simulink model "ironCub"  (Simulink 8.6)
settings: Solver=FixedStepAuto  StartTime=0.0  StopTime=config.simulationTime  FixedStep=config.Ts  RelTol=1e-3
InitFcn:
  | cd(fileparts(which(bdroot)));
  | initIronCub;
StopFcn:
  | visualizer_demo(time.Data,state.Data,config,desired_x_dx_ddx_dddx_CoM,jetsIntensitiesByWeight);
values from neighbouring files (symbols this model uses):
  config = struct    [initIronCub.m]
  ROBOT_DOF = config.ndof    [initIronCub.m]
libraries: WBToolboxLibrary x99
(part 2 of 2)

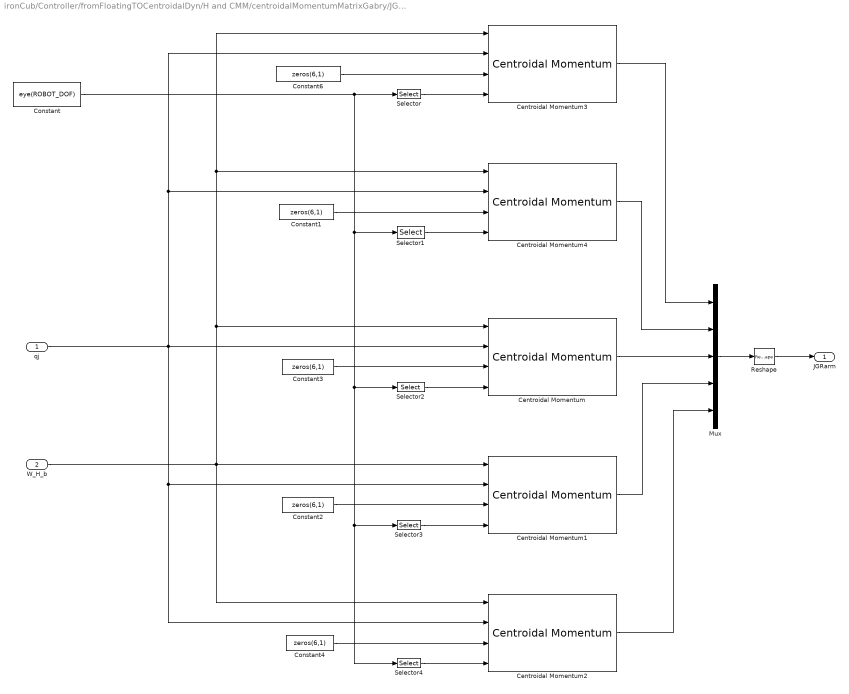
== system ironCub/Controller/fromFloatingTOCentroidalDyn/H and CMM/centroidalMomentumMatrixGabry/JGjoints/JGRarm ==
  qj : Inport
  W_H_b : Inport  Port=2
  Centroidal Momentum{,1..4} (5 alike) : WBToolboxLibrary/wholeBodyModel/Dynamics/Centroidal Momentum  robotName=WBT_robotName  localName=WBT_modelName  wbiFile=WBT_wbiFilename  wbiList=WBT_wbiList
  Constant : Constant  Value=eye(ROBOT_DOF)
  Constant{1..4,6} (5 alike) : Constant  Value=zeros(6,1)
  Mux : Mux  Inputs=5
  Reshape : Reshape  OutputDimensionality=Customize  OutputDimensions=[6,5]
  Selector : Selector  NumberOfDimensions=2  InputPortWidth=3  IndexOptions=Index vector (dialog),Select all  Indices=[9],1  OutputSizes=1,1
  Selector1 : Selector  NumberOfDimensions=2  InputPortWidth=3  IndexOptions=Index vector (dialog),Select all  Indices=[10],1  OutputSizes=1,1
  Selector2 : Selector  NumberOfDimensions=2  InputPortWidth=3  IndexOptions=Index vector (dialog),Select all  Indices=[11],1  OutputSizes=1,1
  Selector3 : Selector  NumberOfDimensions=2  InputPortWidth=3  IndexOptions=Index vector (dialog),Select all  Indices=[12],1  OutputSizes=1,1
  Selector4 : Selector  NumberOfDimensions=2  InputPortWidth=3  IndexOptions=Index vector (dialog),Select all  Indices=[13],1  OutputSizes=1,1
  JGRarm : Outport
  wires:
  Constant6/1 -> Centroidal Momentum3/3
  Constant1/1 -> Centroidal Momentum4/3
  Constant3/1 -> Centroidal Momentum/3
  Constant4/1 -> Centroidal Momentum2/3
  Constant2/1 -> Centroidal Momentum1/3
  qj/1 -> Centroidal Momentum4/2, Centroidal Momentum3/2, Centroidal Momentum2/2, Centroidal Momentum1/2, Centroidal Momentum/2
  W_H_b/1 -> Centroidal Momentum1/1, Centroidal Momentum2/1, Centroidal Momentum/1, Centroidal Momentum3/1, Centroidal Momentum4/1
  Constant/1 -> Selector4/1, Selector3/1, Selector2/1, Selector1/1, Selector/1
  Selector/1 -> Centroidal Momentum3/4
  Selector1/1 -> Centroidal Momentum4/4
  Selector2/1 -> Centroidal Momentum/4
  Selector3/1 -> Centroidal Momentum1/4
  Selector4/1 -> Centroidal Momentum2/4
  Centroidal Momentum/1 -> Mux/3
  Centroidal Momentum3/1 -> Mux/1
  Centroidal Momentum4/1 -> Mux/2
  Centroidal Momentum1/1 -> Mux/4
  Centroidal Momentum2/1 -> Mux/5
  Mux/1 -> Reshape/1
  Reshape/1 -> JGRarm/1

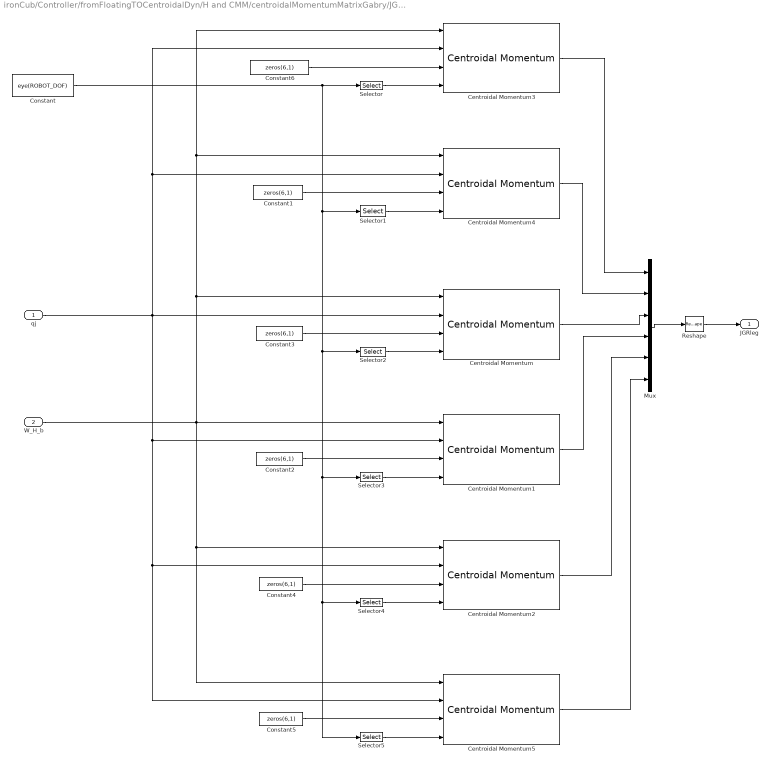
== system ironCub/Controller/fromFloatingTOCentroidalDyn/H and CMM/centroidalMomentumMatrixGabry/JGjoints/JGRleg ==
  qj : Inport
  W_H_b : Inport  Port=2
  Centroidal Momentum{,1..5} (6 alike) : WBToolboxLibrary/wholeBodyModel/Dynamics/Centroidal Momentum  robotName=WBT_robotName  localName=WBT_modelName  wbiFile=WBT_wbiFilename  wbiList=WBT_wbiList
  Constant : Constant  Value=eye(ROBOT_DOF)
  Constant{1..6} (6 alike) : Constant  Value=zeros(6,1)
  Mux : Mux  Inputs=6
  Reshape : Reshape  OutputDimensionality=Customize  OutputDimensions=[6,6]
  Selector : Selector  NumberOfDimensions=2  InputPortWidth=3  IndexOptions=Index vector (dialog),Select all  Indices=[20],1  OutputSizes=1,1
  Selector1 : Selector  NumberOfDimensions=2  InputPortWidth=3  IndexOptions=Index vector (dialog),Select all  Indices=[21],1  OutputSizes=1,1
  Selector2 : Selector  NumberOfDimensions=2  InputPortWidth=3  IndexOptions=Index vector (dialog),Select all  Indices=[22],1  OutputSizes=1,1
  Selector3 : Selector  NumberOfDimensions=2  InputPortWidth=3  IndexOptions=Index vector (dialog),Select all  Indices=[23],1  OutputSizes=1,1
  Selector4 : Selector  NumberOfDimensions=2  InputPortWidth=3  IndexOptions=Index vector (dialog),Select all  Indices=[24],1  OutputSizes=1,1
  Selector5 : Selector  NumberOfDimensions=2  InputPortWidth=3  IndexOptions=Index vector (dialog),Select all  Indices=[25],1  OutputSizes=1,1
  JGRleg : Outport
  wires:
  Constant6/1 -> Centroidal Momentum3/3
  Constant1/1 -> Centroidal Momentum4/3
  Constant3/1 -> Centroidal Momentum/3
  Constant4/1 -> Centroidal Momentum2/3
  Constant2/1 -> Centroidal Momentum1/3
  qj/1 -> Centroidal Momentum4/2, Centroidal Momentum3/2, Centroidal Momentum5/2, Centroidal Momentum2/2, Centroidal Momentum1/2, Centroidal Momentum/2
  W_H_b/1 -> Centroidal Momentum1/1, Centroidal Momentum5/1, Centroidal Momentum2/1, Centroidal Momentum/1, Centroidal Momentum3/1, Centroidal Momentum4/1
  Selector/1 -> Centroidal Momentum3/4
  Selector1/1 -> Centroidal Momentum4/4
  Selector2/1 -> Centroidal Momentum/4
  Selector3/1 -> Centroidal Momentum1/4
  Selector4/1 -> Centroidal Momentum2/4
  Centroidal Momentum/1 -> Mux/3
  Centroidal Momentum3/1 -> Mux/1
  Centroidal Momentum4/1 -> Mux/2
  Centroidal Momentum1/1 -> Mux/4
  Centroidal Momentum2/1 -> Mux/5
  Mux/1 -> Reshape/1
  Reshape/1 -> JGRleg/1
  Constant5/1 -> Centroidal Momentum5/3
  Constant/1 -> Selector5/1, Selector4/1, Selector3/1, Selector2/1, Selector1/1, Selector/1
  Selector5/1 -> Centroidal Momentum5/4
  Centroidal Momentum5/1 -> Mux/6

== system ironCub/Controller/fromFloatingTOCentroidalDyn/H and CMM/centroidalMomentumMatrixGabry/JGjoints/JGtorso ==
  qj : Inport
  W_H_b : Inport  Port=2
  Centroidal Momentum : WBToolboxLibrary/wholeBodyModel/Dynamics/Centroidal Momentum  robotName=WBT_robotName  localName=WBT_modelName  wbiFile=WBT_wbiFilename  wbiList=WBT_wbiList
  Centroidal Momentum3 : WBToolboxLibrary/wholeBodyModel/Dynamics/Centroidal Momentum  robotName=WBT_robotName  localName=WBT_modelName  wbiFile=WBT_wbiFilename  wbiList=WBT_wbiList
  Centroidal Momentum4 : WBToolboxLibrary/wholeBodyModel/Dynamics/Centroidal Momentum  robotName=WBT_robotName  localName=WBT_modelName  wbiFile=WBT_wbiFilename  wbiList=WBT_wbiList
  Constant : Constant  Value=eye(ROBOT_DOF)
  Constant1 : Constant  Value=zeros(6,1)
  Constant3 : Constant  Value=zeros(6,1)
  Constant6 : Constant  Value=zeros(6,1)
  Mux : Mux  Inputs=3
  Reshape : Reshape  OutputDimensionality=Customize  OutputDimensions=[6,3]
  Selector : Selector  NumberOfDimensions=2  InputPortWidth=3  IndexOptions=Index vector (dialog),Select all  Indices=[1],1  OutputSizes=1,1
  Selector1 : Selector  NumberOfDimensions=2  InputPortWidth=3  IndexOptions=Index vector (dialog),Select all  Indices=[2],1  OutputSizes=1,1
  Selector2 : Selector  NumberOfDimensions=2  InputPortWidth=3  IndexOptions=Index vector (dialog),Select all  Indices=[3],1  OutputSizes=1,1
  JGtorso : Outport
  wires:
  qj/1 -> Centroidal Momentum3/2, Centroidal Momentum4/2, Centroidal Momentum/2
  W_H_b/1 -> Centroidal Momentum/1, Centroidal Momentum4/1, Centroidal Momentum3/1
  Centroidal Momentum3/1 -> Mux/1
  Centroidal Momentum4/1 -> Mux/2
  Centroidal Momentum/1 -> Mux/3
  Constant6/1 -> Centroidal Momentum3/3
  Constant1/1 -> Centroidal Momentum4/3
  Constant3/1 -> Centroidal Momentum/3
  Mux/1 -> Reshape/1
  Constant/1 -> Selector2/1, Selector1/1, Selector/1
  Selector/1 -> Centroidal Momentum3/4
  Selector1/1 -> Centroidal Momentum4/4
  Selector2/1 -> Centroidal Momentum/4
  Reshape/1 -> JGtorso/1

== matlab function Controller/stateDemuxFCN ==
  data: state input double; basePose output double; jointAngles output double; baseVelocity output double; jointsVelocity output double; config parameter double
function [basePose,jointAngles,baseVelocity,jointsVelocity] = stateDemuxFCN(state,config)
%#codegen
    
    [basePose,jointAngles,baseVelocity,jointsVelocity] = stateDemux(state,config);
end

== matlab function Controller/comRefs/trajectoryGeneratorCoM ==
  data: t input double; CoM0 input double; w_H_b0 input double; comDes output double; config parameter double; rotBaseDes output double; xDcomDes output double; tSettling output double
function [comDes,rotBaseDes,xDcomDes,tSettling]  = referencesFCN(t,CoM0,w_H_b0,config)
%#codegen

[comDes,rotBaseDes,xDcomDes,tSettling]  = references(t,CoM0,w_H_b0,config);

== matlab function Dynamics/Subsystem/kinematicsFCN ==
  data: jointVels input double; state input double; stateDot output double; config parameter double
function stateDot = kinematicsFCN(jointVels,state,config)
%#codegen

    stateDot = kinematics(jointVels,state,config);
end

== matlab function Controller/transpose ==
  data: u input double; uTranspose output double
function uTranspose = transpose(u)
%#codegen
uTranspose = u';

== matlab function Controller/controller/controllerFlyingHumanoidsFCN ==
  data: jetsIntensities input double; matrixOfJetsAxes input double; matrixOfJetsArms input double; w_H_b input double; s input double; sDes input double; Min input double; hin input double; Jin input double; Jcom input double; JDotNu input double; nuin input double; xcom input double; H input double; intH input double; CMMin input double; comRefs input double; baseRotRefs input double; hessianMatrixQP output double; gVectorQP output double; constraintMatA output double; lowerBoundQPMatA output double; upperBoundQPMatA output double; lowerBoundQP output double; upperBoundQP output double; config parameter double; aux output double
function [hessianMatrixQP,gVectorQP,constraintMatA,lowerBoundQPMatA,upperBoundQPMatA,lowerBoundQP,upperBoundQP,aux] = controllerFCN(jetsIntensities,matrixOfJetsAxes,matrixOfJetsArms,w_H_b,s,sDes,Min,hin,Jin,Jcom,JDotNu,nuin,xcom,H,intH,CMMin,comRefs,baseRotRefs,config)
%#codegen

    [hessianMatrixQP,gVectorQP,constraintMatA,lowerBoundQPMatA,upperBoundQPMatA,lowerBoundQP,upperBoundQP,aux] = controller(jetsIntensities,matrixOfJetsAxes,matrixOfJetsArms,w_H_b,s,sDes,Min,hin,Jin,Jcom,JDotNu,nuin,xcom,H,intH,CMMin,comRefs,baseRotRefs,config);
end

== matlab function Dynamics/fromStateToForces/matrixOfJetsAxes/stateDemuxFCN ==
  data: w_H_J1 input double; matrixOfJetsAxes output double; w_H_J2 input double; w_H_J3 input double; w_H_J4 input double; com input double; matrixOfJetsArms output double; config parameter double
function [matrixOfJetsAxes,matrixOfJetsArms] = axesOfJetsFCN(w_H_J1,w_H_J2,w_H_J3,w_H_J4,com,config)
%#codegen

    [matrixOfJetsAxes,matrixOfJetsArms] = axesOfJets(w_H_J1,w_H_J2,w_H_J3,w_H_J4,com,config);
end

== matlab function Controller/controller/torqueControl ==
  data: jetsIntensities input double; matrixOfJetsAxes input double; jointVelDes input double; Min input double; hin input double; Jin input double; nuin input double; intsTildeDot input double; jointTorques output double; config parameter double; jointVelError output double
function [jointTorques,jointVelError] = torqueControlFCN(jetsIntensities,matrixOfJetsAxes,jointVelDes,Min,hin,Jin,nuin,intsTildeDot,config)
%#codegen

    [jointTorques,jointVelError] = torqueControl(jetsIntensities,matrixOfJetsAxes,jointVelDes,Min,hin,Jin,nuin,intsTildeDot,config);
end

== matlab function Controller/transpose1 ==
  data: momentum input double; w_H_b input double; rotBaseDes input double; orientationError output double; config parameter double; angularMomentum output double
function [orientationError, angularMomentum] = norm(momentum,w_H_b,rotBaseDes,config)
%#codegen

    orientationError = norm(rotBaseDes(1:3,1:3)'*w_H_b(1:3,1:3)-eye(3));
    angularMomentum = norm(momentum(4:6));

== matlab function Dynamics/dyanmicsFCN  ==
  data: M input double; h input double; J input double; f input double; tau input double; state input double; stateDot output double; config parameter double
function stateDot = dynamicsFCN(M,h,J,f,tau,state,config)
%#codegen

    stateDot = dynamics(M,h,J,f,tau,state,config);
end

== matlab function Dynamics/fromStateToForces/fromJetsIntensitiesToForces ==
  data: matrixOfJetsAxes input double; jetsIntensities input double; f output double
function f = fromJetsIntensitiesToForcesFCN(matrixOfJetsAxes,jetsIntensities)
%#codegen

    f = fromJetsIntensitiesToForces(matrixOfJetsAxes,jetsIntensities);

end

== matlab function Controller/matrixOfJetsAxes1/stateDemuxFCN ==
  data: w_H_J1 input double; matrixOfJetsAxes output double; w_H_J2 input double; w_H_J3 input double; w_H_J4 input double; com input double; matrixOfJetsArms output double; config parameter double
function [matrixOfJetsAxes,matrixOfJetsArms] = axesOfJetsFCN(w_H_J1,w_H_J2,w_H_J3,w_H_J4,com,config)
%#codegen

    [matrixOfJetsAxes,matrixOfJetsArms] = axesOfJets(w_H_J1,w_H_J2,w_H_J3,w_H_J4,com,config);
end

== matlab function Dynamics/stateDemuxFCN ==
  data: state input double; basePose output double; jointAngles output double; baseVelocity output double; jointsVelocity output double; config parameter double
function [basePose,jointAngles,baseVelocity,jointsVelocity] = stateDemuxFCN(state,config)
%#codegen

    [basePose,jointAngles,baseVelocity,jointsVelocity] = stateDemux(state,config);
end

== matlab function Dynamics/Subsystem/stateDemuxFCN1 ==
  data: state input double; basePose output double; jointAngles output double; baseVelocity output double; jointsVelocity output double; config parameter double
function [basePose,jointAngles,baseVelocity,jointsVelocity] = stateDemuxFCN(state,config)
%#codegen
    [~,jointAngles,baseVelocity,jointsVelocity] = stateDemux(state,config);
    basePose  = state(1:7); 
      
    % state(1:3)  =  I_p_b,     i.e. base position w.r.t. inertial frame
    % state(4:7)  =  Q_b,       i.e. quaternion representing base orientation w.r.t. base frame. More precisely, dot(Q_b) = -0.5 SB(b_omega_b)Q_b
end

== matlab function Controller/controller/Evaluate initial jets intensities ==
  data: matrixOfJetsAxes input double; Min input double; Jin input double; comRefs input double; j0 output double; config parameter double
function   j0 = jetIntensitiesAtZeroFCN(matrixOfJetsAxes,Min,Jin,comRefs,config)
%#codegen

    j0 = jetIntensitiesAtZero(matrixOfJetsAxes,Min,Jin,comRefs,config);
end

== matlab function Controller/controller/transpose1 ==
  data: u input double; normU output double
function normU = norm(u)
%#codegen

normU = norm(u);

== matlab function Controller/fromFloatingTOCentroidalDyn/fromFloating2Centroidal ==
  data: M input double; M_c output double; h input double; g input double; J input double; dJcNu input double; Nu input double; c_T_b input double; dT input double; h_c output double; Jc_c output double; Jc_cDNu_c output double; Nu_c output double; CMM output double; CMMc output double
function [M_c,h_c, Jc_c, Jc_cDNu_c, Nu_c,CMM,CMMc] = fromFloatingToCentroidalDynamicsFCN(M, h, g, J, dJcNu, Nu, c_T_b, dT)
%#codegen
[M_c,h_c, Jc_c, Jc_cDNu_c, Nu_c,CMM,CMMc] = fromFloatingToCentroidalDynamics(M, h, g, J, dJcNu, Nu, c_T_b, dT);

== matlab function Controller/fromFloatingTOCentroidalDyn/fromState2TandTD ==
  data: M input double; xcom input double; c_T_b output double; wHb input double; dxcom input double; dx_b input double; dT output double
function [c_T_b, dT] = centroidalTransformationT_TDot(M,xcom,wHb,dxcom,dx_b)
%#codegen
[c_T_b, dT] = centroidalTransformationT_TDot(xcom,wHb(1:3,4),dxcom,dx_b,M);
